simulink model "bpsk_rx2"  (R2021b)
settings: Solver=VariableStepAuto  StartTime=0.0  StopTime=1000  RelTol=1e-3
libraries: dsp_blocks x7
settings Model: Creator=aidynardabek  LastModifiedBy=aidynardabek

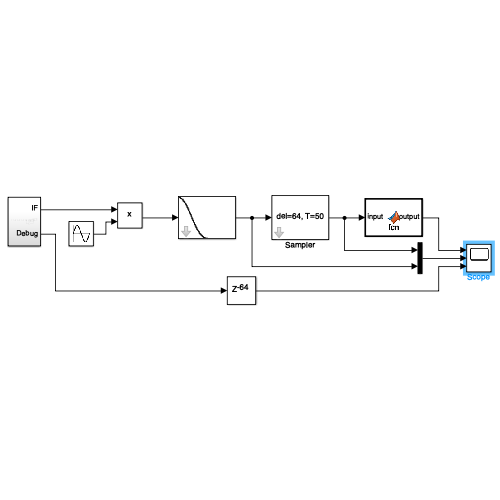
[thumbnail: Simulink's stored preview of the top-level diagram]
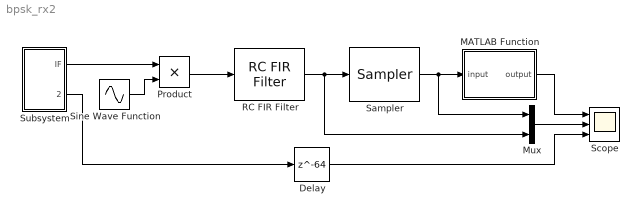
== system bpsk_rx2 ==
  Delay : Delay  DelayLength=64  InitialCondition=0
  MATLAB Function : MATLAB Function  TreatAsAtomicUnit=on
  Mux : Mux  Inputs=2
  Product : Product
  RC FIR Filter : dsp_blocks/Filters/RC FIR Filter  period=50  beta=0.5  root=off  filt_len=128  win_type=on
  Sampler : dsp_blocks/Conversions/Sampler  offset=64  samp_period=50
  Scope : Scope  NumInputPorts=3
  Sine Wave Function : Sin  Amplitude=2  Frequency=2*pi*0.1  SampleTime=0
  Subsystem : Subsystem
  wires:
  Subsystem/1(IF) -> Product/1
  Sine Wave Function/1 -> Product/2
  Subsystem/2(Debug) -> Delay/1
  Product/1 -> RC FIR Filter/1
  RC FIR Filter/1 -> Mux/2, Sampler/1
  Sampler/1 -> Mux/1, MATLAB Function/1(input)
  MATLAB Function/1(output) -> Scope/1
  Delay/1 -> Scope/3
  Mux/1 -> Scope/2

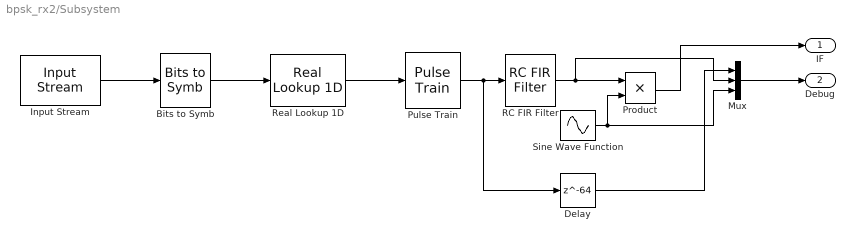
== system bpsk_rx2/Subsystem ==
  Bits to Symb : dsp_blocks/Conversions/Bits to Symb
  Delay : Delay  DelayLength=64
  Input Stream : dsp_blocks/Sources//Sinks/Input Stream  period=50  width=1  fname=rand.mat
  Mux : Mux  Inputs=3
  Product : Product
  Pulse Train : dsp_blocks/Conversions/Pulse Train  period=50
  RC FIR Filter : dsp_blocks/Filters/RC FIR Filter  period=50  beta=0.5  root=off  filt_len=128  win_type=on
  Real Lookup 1D : dsp_blocks/Conversions/Real Lookup 1D  table=[-1 1]
  Sine Wave Function : Sin  Frequency=2*pi*0.1  SampleTime=0
  IF : Outport
  Debug : Outport  Port=2
  wires:
  Delay/1 -> Mux/1
  Mux/1 -> Debug/1
  Bits to Symb/1 -> Real Lookup 1D/1
  RC FIR Filter/1 -> Mux/2, Product/1
  Input Stream/1 -> Bits to Symb/1
  Real Lookup 1D/1 -> Pulse Train/1
  Sine Wave Function/1 -> Mux/3, Product/2
  Product/1 -> IF/1
  Pulse Train/1 -> Delay/1, RC FIR Filter/1

== matlab function bpsk_rx2/MATLAB Function ==
  data: input input; output output
function output = fcn(input)

if (input > 0)
    output = 1;
else
    output = 0;
end
